simulink model "HHEA_Sandbox"  (R2024b)
settings: Solver=VariableStepAuto  StartTime=0.0  StopTime=10.0  RelTol=1e-3
values from neighbouring files (symbols this model uses):
  Ki = -2*pi/5*imag(1/H(1)')    [BranchAndBound.m]    (also in Optimization.m; Parameters.m = 1; RectangularOptimization.m; RoundingPI.m)
  Kp = real(1/H(1)')    [BranchAndBound.m]    (also in Optimization.m; Parameters.m = 2154400; RectangularOptimization.m; RoundingPI.m)
  params = struct    [BranchAndBound.m]    (also in Optimization.m; Parameters.m = struct(); RectangularOptimization.m; RoundingPI.m)
  valveTransferFunction = tf(4/valveSettlingTime,[1 4/valveSettlingTime])    [Parameters.m]
settings Model: Creator=jackson  LastModifiedBy=jackson

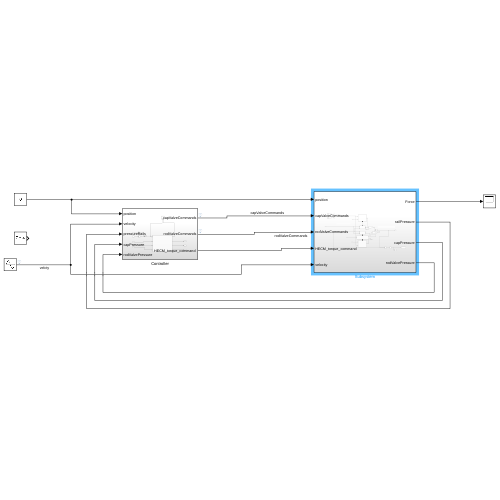
[thumbnail: Simulink's stored preview of the top-level diagram]
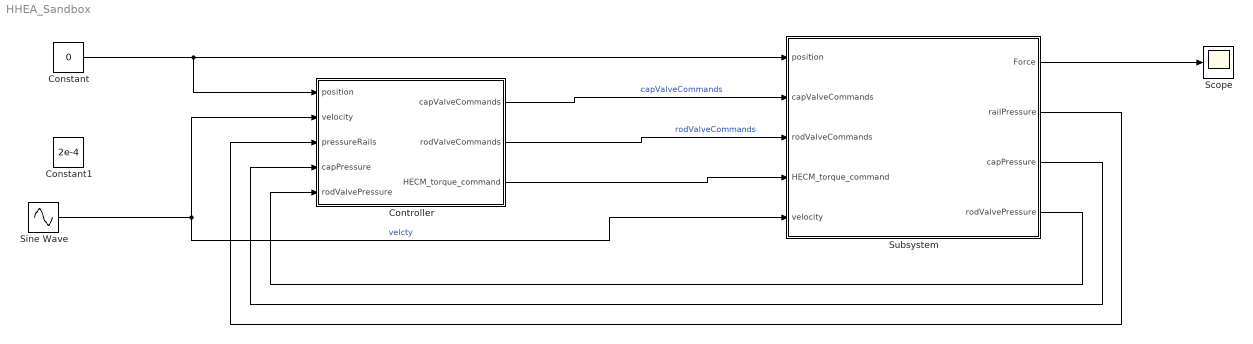
== system HHEA_Sandbox ==
  Constant : Constant  Value=0
  Constant1 : Constant  Value=2e-4
  Controller : Subsystem
  Scope : Scope
  Sine Wave : Sin  SampleTime=0
  Subsystem : Subsystem
  wires:
  Subsystem/4(rodValvePressure) -> Controller/5(rodValvePressure)
  Sine Wave/1 -> Controller/2(velocity), Subsystem/5(velocity)  "velcty"
  Subsystem/3(capPressure) -> Controller/4(capPressure)
  Subsystem/1(Force) -> Scope/1
  Controller/1(capValveCommands) -> Subsystem/2(capValveCommands)  "capValveCommands"
  Subsystem/2(railPressure) -> Controller/3(pressureRails)
  Controller/2(rodValveCommands) -> Subsystem/3(rodValveCommands)  "rodValveCommands"
  Constant/1 -> Controller/1(position), Subsystem/1(position)
  Controller/3("HECM_torque_command ") -> Subsystem/4("HECM_torque_command ")

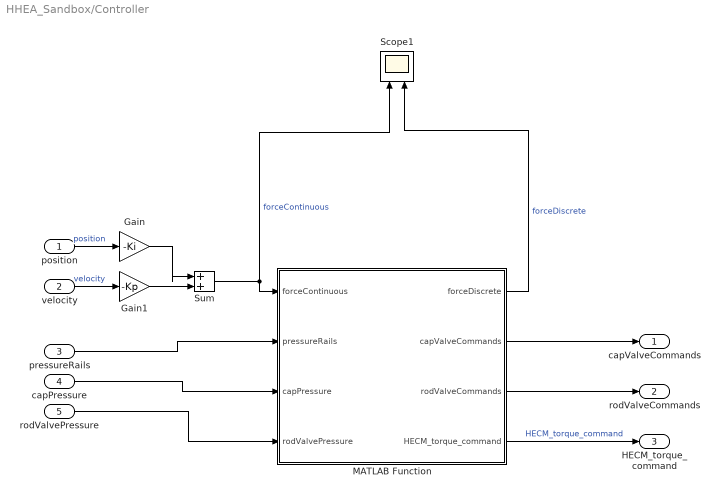
== system HHEA_Sandbox/Controller ==
  position : Inport
  velocity : Inport  Port=2
  pressureRails : Inport  Port=3
  capPressure : Inport  Port=4
  rodValvePressure : Inport  Port=5
  Gain : Gain  Gain=-Ki
  Gain1 : Gain  Gain=-Kp
  MATLAB Function : MATLAB Function  TreatAsAtomicUnit=on
  Scope1 : Scope  NumInputPorts=2
  Sum : Sum  Inputs=|++
  capValveCommands : Outport
  rodValveCommands : Outport  Port=2
  "HECM_torque_command " : Outport  Port=3
  wires:
  velocity/1 -> Gain1/1  "velocity"
  Gain1/1 -> Sum/2
  Gain/1 -> Sum/1
  Sum/1 -> Scope1/1, MATLAB Function/1(forceContinuous)  "forceContinuous"
  MATLAB Function/1(forceDiscrete) -> Scope1/2  "forceDiscrete"
  position/1 -> Gain/1  "position"
  MATLAB Function/2(capValveCommands) -> capValveCommands/1
  MATLAB Function/3(rodValveCommands) -> rodValveCommands/1
  pressureRails/1 -> MATLAB Function/2(pressureRails)
  MATLAB Function/4(HECM_torque_command) -> "HECM_torque_command "/1  "HECM_torque_command"
  capPressure/1 -> MATLAB Function/3(capPressure)
  rodValvePressure/1 -> MATLAB Function/4(rodValvePressure)

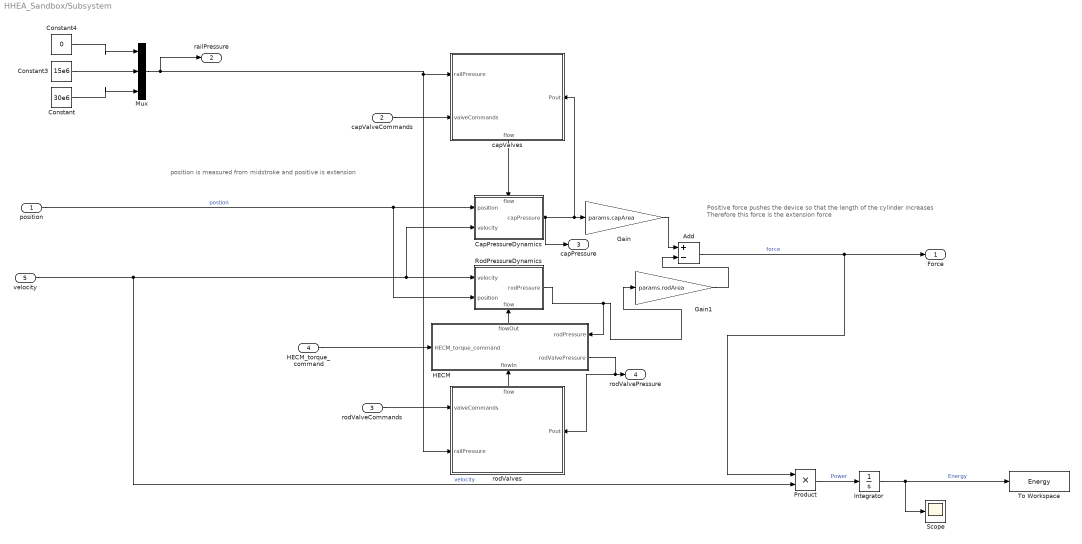
== system HHEA_Sandbox/Subsystem ==
  note: position is measured from midstroke and positive is extension
  note: Positive force pushes the device so that the length of the cylinder increases
      | Therefore this force is the extension force
  position : Inport
  capValveCommands : Inport  Port=2
  rodValveCommands : Inport  Port=3
  "HECM_torque_command " : Inport  Port=4
  velocity : Inport  Port=5
  Add : Sum  Inputs=+-
  CapPressureDynamics : Subsystem
      settings: PortSchema="{\"entries\":[{\"content\":{\"sides\":[{\"content\":{\"connectorIds\":[\"In1\",\"In2\"]},\"type\":\"ConnectorPlacement.EquallySpacedRectSide\",\"uuid\":\"0a444e4d-7364-44e5-8b72-8c210fabafa0\"},{\"content\":{\"connectorIds\":[\"Out1\"],\"side\":\"RIGHT\"},\"type\":\"ConnectorPlacement.EquallySpacedRectSide\",\"uuid\":\"a3669697-8e2e-4fce-83e7-11feb3c41a11\"},{\"content\":{\"connectorIds\":[\"In3\"],\"side\":\"TOP\"},\"type\":\"ConnectorPlacement.EquallySpacedRectSide\",\"uuid\":\"edbd7469-179d-4b36-ab80-dceaa86ef763\"},{\"content\":{\"side\":\"BOTTOM\"},\"type\":\"ConnectorPlacement.EquallySpacedRectSide\",\"uuid\":\"36ba3990-6628-4e3d-ab1a-10917dd4fa0b\"}]},\"type\":\"ConnectorPlacement.EquallySpacedConnector\",\"uuid\":\"68480e3c-12c2-4c1a-9580-60c15ea9a162\"}],\"packageUris\":[\"http://schema.mathworks.com/mf0/Connector/R2020b\"],\"version\":\"1.0\"}"
  Constant : Constant  Value=30e6
  Constant3 : Constant  Value=15e6
  Constant4 : Constant  Value=0
  Gain : Gain  Gain=params.capArea
  Gain1 : Gain  Gain=params.rodArea
  HECM : Subsystem
      settings: PortSchema="{\"entries\":[{\"content\":{\"sides\":[{\"content\":{\"connectorIds\":[\"In1\"]},\"type\":\"ConnectorPlacement.EquallySpacedRectSide\",\"uuid\":\"fa7e009b-3a28-4dd3-907b-76d8fd1f2fc5\"},{\"content\":{\"connectorIds\":[\"Out1\"],\"side\":\"RIGHT\"},\"type\":\"ConnectorPlacement.EquallySpacedRectSide\",\"uuid\":\"b4b71eb1-dc67-4897-9f20-563cedc71b8c\"},{\"content\":{\"connectorIds\":[\"In2\"],\"side\":\"TOP\"},\"type\":\"ConnectorPlacement.EquallySpacedRectSide\",\"uuid\":\"a67ddf4c-e1a7-4a41-beba-4c9482bc4896\"},{\"content\":{\"connectorIds\":[\"Out2\",\"In3\"],\"side\":\"BOTTOM\"},\"type\":\"ConnectorPlacement.EquallySpacedRectSide\",\"uuid\":\"d70e9d30-0c3d-4fe1-994c-11171af7a54f\"}]},\"type\":\"ConnectorPlacement.EquallySpacedConnector\",\"uuid\":\"d5f93414-5adb-4b46-aa3e-a0fd5f50c915\"}],\"packageUris\":[\"http://schema.mathworks.com/mf0/Connector/R2020b\"],\"version\":\"1.0\"}"
  Integrator : Integrator
  Mux : Mux  Inputs=3
  Product : Product
  RodPressureDynamics : Subsystem
      settings: PortSchema="{\"entries\":[{\"content\":{\"sides\":[{\"content\":{\"connectorIds\":[\"In1\",\"In2\"]},\"type\":\"ConnectorPlacement.EquallySpacedRectSide\",\"uuid\":\"0a444e4d-7364-44e5-8b72-8c210fabafa0\"},{\"content\":{\"connectorIds\":[\"Out1\"],\"side\":\"RIGHT\"},\"type\":\"ConnectorPlacement.EquallySpacedRectSide\",\"uuid\":\"a3669697-8e2e-4fce-83e7-11feb3c41a11\"},{\"content\":{\"side\":\"TOP\"},\"type\":\"ConnectorPlacement.EquallySpacedRectSide\",\"uuid\":\"edbd7469-179d-4b36-ab80-dceaa86ef763\"},{\"content\":{\"connectorIds\":[\"In3\"],\"side\":\"BOTTOM\"},\"type\":\"ConnectorPlacement.EquallySpacedRectSide\",\"uuid\":\"0057cc85-602f-4ff7-8e06-c43254199496\"}]},\"type\":\"ConnectorPlacement.EquallySpacedConnector\",\"uuid\":\"68480e3c-12c2-4c1a-9580-60c15ea9a162\"}],\"packageUris\":[\"http://schema.mathworks.com/mf0/Connector/R2020b\"],\"version\":\"1.0\"}"
  Scope : Scope
  To Workspace : ToWorkspace  VariableName=Energy  SampleTime=-1
      settings: MaxDataPoints=1
  capValves : Subsystem
      settings: PortSchema="{\"entries\":[{\"content\":{\"sides\":[{\"content\":{\"connectorIds\":[\"In1\",\"In2\"]},\"type\":\"ConnectorPlacement.EquallySpacedRectSide\",\"uuid\":\"d2e8cfa0-a0ae-49da-8fda-082dfd3b2d9f\"},{\"content\":{\"connectorIds\":[\"In3\"],\"side\":\"RIGHT\"},\"type\":\"ConnectorPlacement.EquallySpacedRectSide\",\"uuid\":\"7b83af61-76d6-4e35-9365-fafdba130762\"},{\"content\":{\"side\":\"TOP\"},\"type\":\"ConnectorPlacement.EquallySpacedRectSide\",\"uuid\":\"6880d985-ed9d-415d-a1a9-fc8aaf1ae9e0\"},{\"content\":{\"connectorIds\":[\"Out1\"],\"side\":\"BOTTOM\"},\"type\":\"ConnectorPlacement.EquallySpacedRectSide\",\"uuid\":\"f70b92c7-c6bf-4dbf-a331-364ba55ce8fb\"}]},\"type\":\"ConnectorPlacement.EquallySpacedConnector\",\"uuid\":\"7ffcaf2b-fb7f-4cb0-b739-43ebea45fc90\"}],\"packageUris\":[\"http://schema.mathworks.com/mf0/Connector/R2020b\"],\"version\":\"1.0\"}"
  rodValves : Subsystem
      settings: PortSchema="{\"entries\":[{\"content\":{\"sides\":[{\"content\":{\"connectorIds\":[\"In1\",\"In2\"]},\"type\":\"ConnectorPlacement.EquallySpacedRectSide\",\"uuid\":\"d2e8cfa0-a0ae-49da-8fda-082dfd3b2d9f\"},{\"content\":{\"connectorIds\":[\"In3\"],\"side\":\"RIGHT\"},\"type\":\"ConnectorPlacement.EquallySpacedRectSide\",\"uuid\":\"7b83af61-76d6-4e35-9365-fafdba130762\"},{\"content\":{\"connectorIds\":[\"Out1\"],\"side\":\"TOP\"},\"type\":\"ConnectorPlacement.EquallySpacedRectSide\",\"uuid\":\"6880d985-ed9d-415d-a1a9-fc8aaf1ae9e0\"},{\"content\":{\"side\":\"BOTTOM\"},\"type\":\"ConnectorPlacement.EquallySpacedRectSide\",\"uuid\":\"f70b92c7-c6bf-4dbf-a331-364ba55ce8fb\"}]},\"type\":\"ConnectorPlacement.EquallySpacedConnector\",\"uuid\":\"7ffcaf2b-fb7f-4cb0-b739-43ebea45fc90\"}],\"packageUris\":[\"http://schema.mathworks.com/mf0/Connector/R2020b\"],\"version\":\"1.0\"}"
  Force : Outport
  railPressure : Outport  Port=2
  capPressure : Outport  Port=3
  rodValvePressure : Outport  Port=4
  wires:
  Gain/1 -> Add/1
  Constant/1 -> Mux/3
  Constant3/1 -> Mux/2
  Gain1/1 -> Add/2
  rodValves/1(flow) -> HECM/1(flowIn)
  capValves/1(flow) -> CapPressureDynamics/3(flow)
  Constant4/1 -> Mux/1
  position/1 -> RodPressureDynamics/2(position), CapPressureDynamics/1(position)  "postion"
  Integrator/1 -> To Workspace/1, Scope/1  "Energy"
  velocity/1 -> Product/2, RodPressureDynamics/1(velocity), CapPressureDynamics/2(velocity)  "velocity"
  capValveCommands/1 -> capValves/2(valveCommands)
  CapPressureDynamics/1(capPressure) -> capPressure/1, capValves/3(Pout), Gain/1
  Product/1 -> Integrator/1  "Power"
  Add/1 -> Force/1, Product/1  "force"
  Mux/1 -> rodValves/2(railPressure), capValves/1(railPressure), railPressure/1
  rodValveCommands/1 -> rodValves/1(valveCommands)
  HECM/1(flowOut) -> RodPressureDynamics/3(flow)
  "HECM_torque_command "/1 -> HECM/2(HECM_torque_command)
  HECM/2(rodValvePressure) -> rodValves/3(Pout), rodValvePressure/1
  RodPressureDynamics/1(rodPressure) -> Gain1/1, HECM/3(rodPressure)

== system HHEA_Sandbox/Subsystem/CapPressureDynamics ==
  position : Inport
  velocity : Inport  Port=2
  flow : Inport  Port=3
  Integrator : Integrator
  MATLAB Function : MATLAB Function  TreatAsAtomicUnit=on
  capPressure : Outport
  wires:
  MATLAB Function/1(pressure_dot) -> Integrator/1
  Integrator/1 -> capPressure/1  "capPressure"
  flow/1 -> MATLAB Function/3(flow)
  velocity/1 -> MATLAB Function/2(velocity)
  position/1 -> MATLAB Function/1(position)

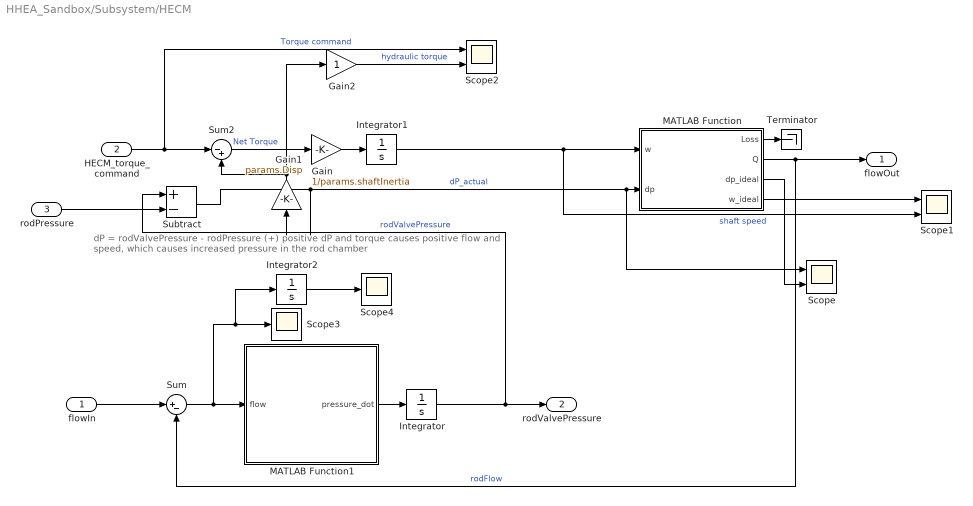
== system HHEA_Sandbox/Subsystem/HECM ==
  note: dP = rodValvePressure - rodPressure
      | (+) positive dP and torque causes positive flow and speed, which causes increased pressure in the rod chamber
  flowIn : Inport
  HECM_torque_command : Inport  Port=2
  rodPressure : Inport  Port=3
  Gain : Gain  Gain=1/params.shaftInertia
  Gain1 : Gain  Gain=params.Disp
  Gain2 : Gain
  Integrator : Integrator
  Integrator1 : Integrator
  Integrator2 : Integrator
  MATLAB Function : MATLAB Function  TreatAsAtomicUnit=on
  MATLAB Function1 : MATLAB Function  TreatAsAtomicUnit=on
  Scope : Scope  NumInputPorts=2
  Scope1 : Scope  NumInputPorts=2
  Scope2 : Scope  NumInputPorts=2
  Scope3 : Scope
  Scope4 : Scope
  Subtract : Sum  Inputs=+-
  Sum : Sum  Inputs=|+-
  Sum2 : Sum  Inputs=|-+
  Terminator : Terminator
  flowOut : Outport
  rodValvePressure : Outport  Port=2
  wires:
  Sum/1 -> Integrator2/1, Scope3/1, MATLAB Function1/1(flow)
  flowIn/1 -> Sum/1
  MATLAB Function1/1(pressure_dot) -> Integrator/1
  Subtract/1 -> Scope/1, MATLAB Function/2(dp), Gain1/1  "dP_actual"
  MATLAB Function/1(Loss) -> Terminator/1
  MATLAB Function/3(dp_ideal) -> Scope/2
  MATLAB Function/4(w_ideal) -> Scope1/1
  Integrator1/1 -> Scope1/2, MATLAB Function/1(w)  "shaft speed"
  HECM_torque_command/1 -> Sum2/1, Scope2/1  "Torque command"
  Sum2/1 -> Gain/1  "Net Torque"
  Gain/1 -> Integrator1/1
  rodPressure/1 -> Subtract/2
  Integrator/1 -> rodValvePressure/1, Subtract/1  "rodValvePressure"
  MATLAB Function/2(Q) -> flowOut/1, Sum/2  "rodFlow"
  Gain1/1 -> Gain2/1, Sum2/2
  Integrator2/1 -> Scope4/1
  Gain2/1 -> Scope2/2  "hydraulic torque"

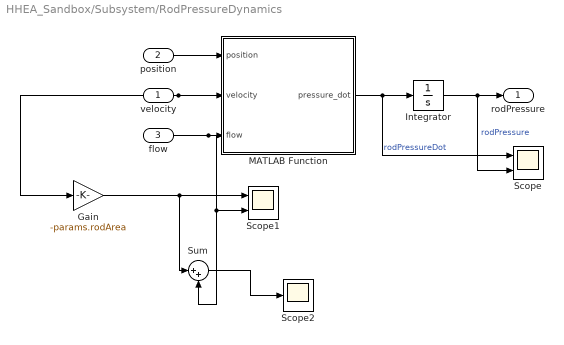
== system HHEA_Sandbox/Subsystem/RodPressureDynamics ==
  velocity : Inport
  position : Inport  Port=2
  flow : Inport  Port=3
  Gain : Gain  Gain=-params.rodArea
  Integrator : Integrator
  MATLAB Function : MATLAB Function  TreatAsAtomicUnit=on
  Scope : Scope  NumInputPorts=2
  Scope1 : Scope  NumInputPorts=2
  Scope2 : Scope
  Sum : Sum  Inputs=|++
  rodPressure : Outport
  wires:
  position/1 -> MATLAB Function/1(position)
  velocity/1 -> MATLAB Function/2(velocity), Gain/1
  flow/1 -> Sum/2, Scope1/2, MATLAB Function/3(flow)
  Integrator/1 -> Scope/2, rodPressure/1  "rodPressure"
  MATLAB Function/1(pressure_dot) -> Scope/1, Integrator/1  "rodPressureDot"
  Gain/1 -> Sum/1, Scope1/1
  Sum/1 -> Scope2/1

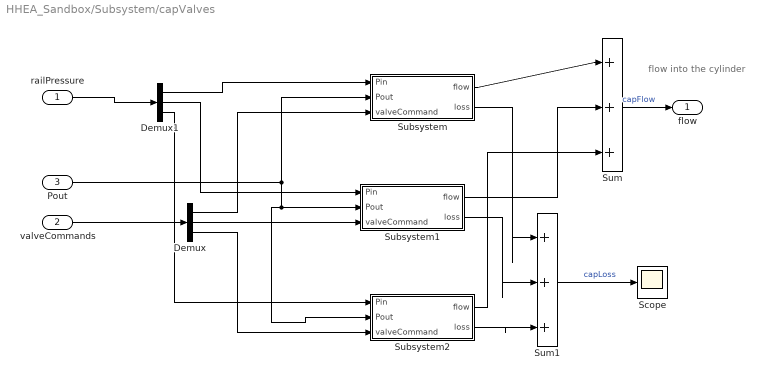
== system HHEA_Sandbox/Subsystem/capValves ==
  note: flow into the cylinder
  railPressure : Inport
  valveCommands : Inport  Port=2
  Pout : Inport  Port=3
  Demux : Demux  Outputs=3
  Demux1 : Demux  Outputs=3
  Scope : Scope
  Subsystem : Subsystem
  Subsystem1 : Subsystem
  Subsystem2 : Subsystem
  Sum : Sum  Inputs=|+++
  Sum1 : Sum  Inputs=|+++
  flow : Outport
  wires:
  Pout/1 -> Subsystem/2(Pout), Subsystem2/2(Pout), Subsystem1/2(Pout)
  valveCommands/1 -> Demux/1
  Demux/1 -> Subsystem/3(valveCommand)
  Demux/2 -> Subsystem1/3(valveCommand)
  Demux/3 -> Subsystem2/3(valveCommand)
  Subsystem/1(flow) -> Sum/1
  Subsystem1/1(flow) -> Sum/2
  Subsystem2/1(flow) -> Sum/3
  Sum/1 -> flow/1  "capFlow"
  Subsystem/2(loss) -> Sum1/1
  Subsystem1/2(loss) -> Sum1/2
  Subsystem2/2(loss) -> Sum1/3
  Sum1/1 -> Scope/1  "capLoss"
  railPressure/1 -> Demux1/1
  Demux1/1 -> Subsystem/1(Pin)
  Demux1/2 -> Subsystem1/1(Pin)
  Demux1/3 -> Subsystem2/1(Pin)

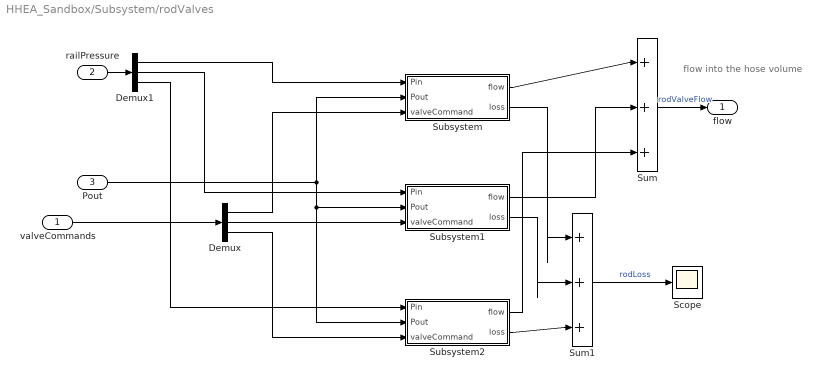
== system HHEA_Sandbox/Subsystem/rodValves ==
  note: flow into the hose volume
  valveCommands : Inport
  railPressure : Inport  Port=2
  Pout : Inport  Port=3
  Demux : Demux  Outputs=3
  Demux1 : Demux  Outputs=3
  Scope : Scope
  Subsystem : Subsystem
  Subsystem1 : Subsystem
  Subsystem2 : Subsystem
  Sum : Sum  Inputs=|+++
  Sum1 : Sum  Inputs=|+++
  flow : Outport
  wires:
  Pout/1 -> Subsystem/2(Pout), Subsystem2/2(Pout), Subsystem1/2(Pout)
  valveCommands/1 -> Demux/1
  Demux/1 -> Subsystem/3(valveCommand)
  Demux1/2 -> Subsystem1/1(Pin)
  Demux1/3 -> Subsystem2/1(Pin)
  Demux/2 -> Subsystem1/3(valveCommand)
  Demux/3 -> Subsystem2/3(valveCommand)
  Subsystem/1(flow) -> Sum/1
  Subsystem1/1(flow) -> Sum/2
  Subsystem2/1(flow) -> Sum/3
  Sum/1 -> flow/1  "rodValveFlow"
  Subsystem/2(loss) -> Sum1/1
  Subsystem1/2(loss) -> Sum1/2
  Subsystem2/2(loss) -> Sum1/3
  Sum1/1 -> Scope/1  "rodLoss"
  railPressure/1 -> Demux1/1
  Demux1/1 -> Subsystem/1(Pin)

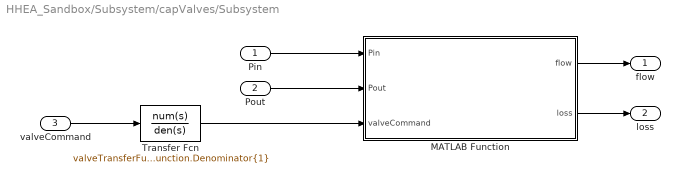
== system HHEA_Sandbox/Subsystem/capValves/Subsystem ==
  Pin : Inport
  Pout : Inport  Port=2
  valveCommand : Inport  Port=3
  MATLAB Function : MATLAB Function  TreatAsAtomicUnit=on
  Transfer Fcn : TransferFcn  Numerator=valveTransferFunction.Numerator{1}  Denominator=valveTransferFunction.Denominator{1}
  flow : Outport
  loss : Outport  Port=2
  wires:
  MATLAB Function/1(flow) -> flow/1
  valveCommand/1 -> Transfer Fcn/1
  Pout/1 -> MATLAB Function/2(Pout)
  Pin/1 -> MATLAB Function/1(Pin)
  MATLAB Function/2(loss) -> loss/1
  Transfer Fcn/1 -> MATLAB Function/3(valveCommand)

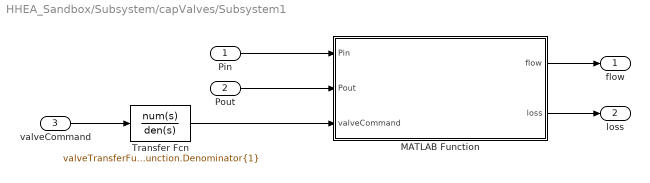
== system HHEA_Sandbox/Subsystem/capValves/Subsystem1 ==
  Pin : Inport
  Pout : Inport  Port=2
  valveCommand : Inport  Port=3
  MATLAB Function : MATLAB Function  TreatAsAtomicUnit=on
  Transfer Fcn : TransferFcn  Numerator=valveTransferFunction.Numerator{1}  Denominator=valveTransferFunction.Denominator{1}
  flow : Outport
  loss : Outport  Port=2
  wires:
  MATLAB Function/1(flow) -> flow/1
  valveCommand/1 -> Transfer Fcn/1
  Pout/1 -> MATLAB Function/2(Pout)
  Pin/1 -> MATLAB Function/1(Pin)
  MATLAB Function/2(loss) -> loss/1
  Transfer Fcn/1 -> MATLAB Function/3(valveCommand)

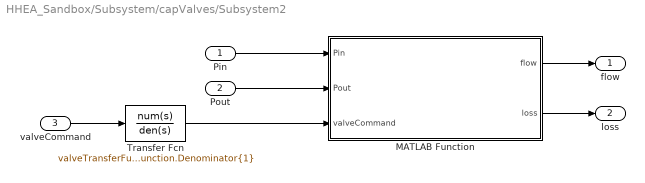
== system HHEA_Sandbox/Subsystem/capValves/Subsystem2 ==
  Pin : Inport
  Pout : Inport  Port=2
  valveCommand : Inport  Port=3
  MATLAB Function : MATLAB Function  TreatAsAtomicUnit=on
  Transfer Fcn : TransferFcn  Numerator=valveTransferFunction.Numerator{1}  Denominator=valveTransferFunction.Denominator{1}
  flow : Outport
  loss : Outport  Port=2
  wires:
  MATLAB Function/1(flow) -> flow/1
  valveCommand/1 -> Transfer Fcn/1
  Pout/1 -> MATLAB Function/2(Pout)
  Pin/1 -> MATLAB Function/1(Pin)
  MATLAB Function/2(loss) -> loss/1
  Transfer Fcn/1 -> MATLAB Function/3(valveCommand)

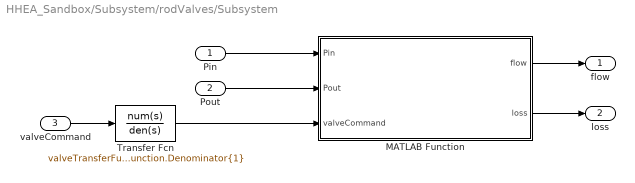
== system HHEA_Sandbox/Subsystem/rodValves/Subsystem ==
  Pin : Inport
  Pout : Inport  Port=2
  valveCommand : Inport  Port=3
  MATLAB Function : MATLAB Function  TreatAsAtomicUnit=on
  Transfer Fcn : TransferFcn  Numerator=valveTransferFunction.Numerator{1}  Denominator=valveTransferFunction.Denominator{1}
  flow : Outport
  loss : Outport  Port=2
  wires:
  MATLAB Function/1(flow) -> flow/1
  valveCommand/1 -> Transfer Fcn/1
  Pout/1 -> MATLAB Function/2(Pout)
  Pin/1 -> MATLAB Function/1(Pin)
  MATLAB Function/2(loss) -> loss/1
  Transfer Fcn/1 -> MATLAB Function/3(valveCommand)

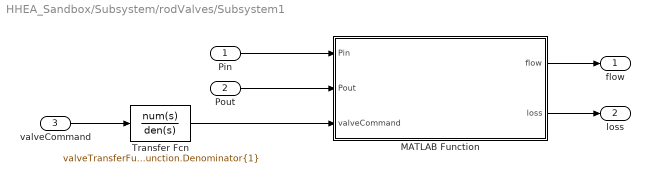
== system HHEA_Sandbox/Subsystem/rodValves/Subsystem1 ==
  Pin : Inport
  Pout : Inport  Port=2
  valveCommand : Inport  Port=3
  MATLAB Function : MATLAB Function  TreatAsAtomicUnit=on
  Transfer Fcn : TransferFcn  Numerator=valveTransferFunction.Numerator{1}  Denominator=valveTransferFunction.Denominator{1}
  flow : Outport
  loss : Outport  Port=2
  wires:
  MATLAB Function/1(flow) -> flow/1
  valveCommand/1 -> Transfer Fcn/1
  Pout/1 -> MATLAB Function/2(Pout)
  Pin/1 -> MATLAB Function/1(Pin)
  MATLAB Function/2(loss) -> loss/1
  Transfer Fcn/1 -> MATLAB Function/3(valveCommand)

== system HHEA_Sandbox/Subsystem/rodValves/Subsystem2 ==
  Pin : Inport
  Pout : Inport  Port=2
  valveCommand : Inport  Port=3
  MATLAB Function : MATLAB Function  TreatAsAtomicUnit=on
  Transfer Fcn : TransferFcn  Numerator=valveTransferFunction.Numerator{1}  Denominator=valveTransferFunction.Denominator{1}
  flow : Outport
  loss : Outport  Port=2
  wires:
  MATLAB Function/1(flow) -> flow/1
  valveCommand/1 -> Transfer Fcn/1
  Pout/1 -> MATLAB Function/2(Pout)
  Pin/1 -> MATLAB Function/1(Pin)
  MATLAB Function/2(loss) -> loss/1
  Transfer Fcn/1 -> MATLAB Function/3(valveCommand)

== matlab function HHEA_Sandbox/Subsystem/rodValves/Subsystem1/MATLAB Function ==
  data: Pin input; flow output; Pout input; valveCommand input; params parameter; loss output
function [flow,loss] = fcn(Pin,Pout,valveCommand,params)
dP = Pin-Pout;
flow = valveCommand*params.valveConstant*sqrt(abs(dP))*sign(dP);
loss = (dP)*flow;

== matlab function HHEA_Sandbox/Subsystem/rodValves/Subsystem2/MATLAB Function ==
  data: Pin input; flow output; Pout input; valveCommand input; params parameter; loss output
function [flow,loss] = fcn(Pin,Pout,valveCommand,params)
dP = Pin-Pout;
flow = valveCommand*params.valveConstant*sqrt(abs(dP))*sign(dP);
loss = (dP)*flow;

== matlab function HHEA_Sandbox/Subsystem/HECM/MATLAB Function1 ==
  data: pressure_dot output; flow input; params parameter
function pressure_dot = RodValvePressure(flow,params)
% This code calculates the pressure dynamics on the rod side of the cylinder
% flow is net flow into the volume from the valves and the actuator

pressure_dot = params.beta/params.hoseVolume*flow;

== matlab function HHEA_Sandbox/Subsystem/HECM/MATLAB Function ==
  data: Loss output; Q output; dp_ideal output; w input; dp input; params parameter; w_ideal output
function [Loss,Q,dp_ideal,w_ideal] = fcn(w,dp,params)
% pump map is loaded in parameters script
% sign convention is that of a pump

T = params.scaleHECM*interp2(params.P1_Mapping,params.w1rad_Mapping,params.T1_Act_Mapping,dp,w);
Q = params.scaleHECM*interp2(params.P1_Mapping,params.w1rad_Mapping,params.Q1_Act_Mapping,dp,w);

Loss = T*w-dp*Q;

% check that it makes sense
D = 107/1e6/2/pi * params.scaleHECM;
dp_ideal = T/D;
w_ideal = Q/D;

== matlab function HHEA_Sandbox/Subsystem/CapPressureDynamics/MATLAB Function ==
  data: position input; velocity input; pressure_dot output; flow input; params parameter
function pressure_dot = CapPressure(position,velocity,flow,params)
% This code calculates the pressure dynamics on the cap side of the cylinder
% flow is flow into the cap side from the valves
% rod side is connected to the flap, positive velocity is extension

%Position is measured from mid stroke. Positive is in extention

volume = params.capArea*(params.cylinderStroke/2 + position);
pressure_dot = params.beta/volume * (flow - velocity*params.capArea);

== matlab function HHEA_Sandbox/Controller/MATLAB Function ==
  data: forceDiscrete output; capValveCommands output; rodValveCommands output; forceContinuous input; pressureRails input; capPressure input; rodValvePressure input; params parameter; HECM_torque_command output
function [forceDiscrete,capValveCommands,rodValveCommands,HECM_torque_command] = fcn(forceContinuous, pressureRails,capPressure,rodValvePressure,params)
%% pressure Rail Commands
% pressureRails = [0; 15; 30]*1e6; % [Pa]
capForce = params.capArea *pressureRails;
rodForce = params.rodArea *pressureRails;

forceOptionsMatrix = capForce' - rodForce;
rodPressure = -1; % initialize
ind = NaN; forceDiscrete = NaN;capValveCommands = zeros(size(pressureRails)); rodValveCommands = zeros(size(pressureRails)); HECM_torque_command = NaN;
while rodPressure < 0
[~,ind] = min(abs(forceOptionsMatrix-forceContinuous),[],'all');
[rodInd,capInd] = ind2sub(size(forceOptionsMatrix),ind);
forceDiscrete = params.capArea *pressureRails(capInd) - params.rodArea *pressureRails(rodInd);

% make bus to send to valves
capValveCommands = zeros(size(pressureRails)); capValveCommands(capInd) = 1;
rodValveCommands = zeros(size(pressureRails)); rodValveCommands(rodInd) = 1;

%% Hecm command
forceDiscreteActual = params.capArea*capPressure - rodValvePressure *params.rodArea;
dP_command = (forceContinuous-forceDiscreteActual) / params.rodArea;
dP_actual = rodValvePressure-rodPressure;
dP_error = dP_command - dP_actual;
HECM_torque_command = .5*dP_error*params.Disp; % proportional controller

rodPressure = rodValvePressure - dP_command;

% assign that entry to NaN for the next loop in case rodPressure is less than zero,
forceOptionsMatrix(ind) = NaN;

end

% check that dP_command gets to the continuous force
[capPressure*params.capArea - rodPressure*params.rodArea, forceContinuous];

== matlab function HHEA_Sandbox/Subsystem/RodPressureDynamics/MATLAB Function ==
  data: position input; velocity input; pressure_dot output; flow input; params parameter
function pressure_dot = RodPressure(position,velocity,flow,params)
% This code calculates the pressure dynamics on the rod side of the cylinder
% flow is flow into the rod side from the valves
% rod side is connected to the flap, positive velocity is extension

% Position is measured from mid stroke. Positive is in extention
volume = params.capArea*( params.cylinderStroke/2 - position);
pressure_dot = params.beta/volume * (flow + velocity*params.rodArea);

== matlab function HHEA_Sandbox/Subsystem/capValves/Subsystem/MATLAB Function ==
  data: Pin input; flow output; Pout input; valveCommand input; params parameter; loss output
function [flow,loss] = fcn(Pin,Pout,valveCommand,params)
dP = Pin-Pout;
flow = valveCommand*params.valveConstant*sqrt(abs(dP))*sign(dP);
loss = (dP)*flow;

== matlab function HHEA_Sandbox/Subsystem/capValves/Subsystem1/MATLAB Function ==
  data: Pin input; flow output; Pout input; valveCommand input; params parameter; loss output
function [flow,loss] = fcn(Pin,Pout,valveCommand,params)
dP = Pin-Pout;
flow = valveCommand*params.valveConstant*sqrt(abs(dP))*sign(dP);
loss = (dP)*flow;

== matlab function HHEA_Sandbox/Subsystem/capValves/Subsystem2/MATLAB Function ==
  data: Pin input; flow output; Pout input; valveCommand input; params parameter; loss output
function [flow,loss] = fcn(Pin,Pout,valveCommand,params)
dP = Pin-Pout;
flow = valveCommand*params.valveConstant*sqrt(abs(dP))*sign(dP);
loss = (dP)*flow;

== matlab function HHEA_Sandbox/Subsystem/rodValves/Subsystem/MATLAB Function ==
  data: Pin input; flow output; Pout input; valveCommand input; params parameter; loss output
function [flow,loss] = fcn(Pin,Pout,valveCommand,params)
dP = Pin-Pout;
flow = valveCommand*params.valveConstant*sqrt(abs(dP))*sign(dP);
loss = (dP)*flow;
